simulink model "van_der_pol"  (R2017b)
settings: Solver=VariableStepAuto  StartTime=0.0  StopTime=10.0  RelTol=1e-3
undefined symbols (not defined in the file): x0, y0
settings Model: Creator=ernst  LastModifiedBy=ernst
settings DataIOCC: SaveFormat=StructureWithTime

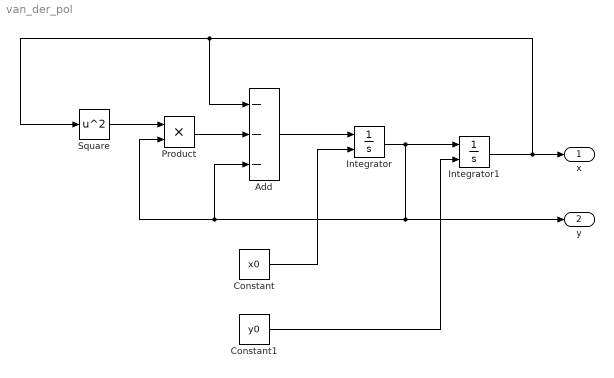
== system van_der_pol ==
  Add : Sum  Inputs=---
  Constant : Constant  Value=x0
  Constant1 : Constant  Value=y0
  Integrator : Integrator  InitialConditionSource=external
  Integrator1 : Integrator  InitialConditionSource=external
  Product : Product
  Square : Math  Operator=square  RndMeth=Zero  SaturateOnIntegerOverflow=on
  x : Outport
  y : Outport  Port=2
  wires:
  Integrator/1 -> Integrator1/1, y/1, Add/3, Product/2
  Integrator1/1 -> Add/1, Square/1, x/1
  Add/1 -> Integrator/1
  Product/1 -> Add/2
  Square/1 -> Product/1
  Constant/1 -> Integrator/2
  Constant1/1 -> Integrator1/2
